simulink model "test_4"  (R2017b)
settings: Solver=VariableStepAuto  StartTime=0.0  StopTime=3  RelTol=1e-3
values from neighbouring files (symbols this model uses):
  Cwy1 = 0.0074    [Parameters (2).m]    (also in Parameters.m)
  Cwy2 = 0.0527    [Parameters (2).m]    (also in Parameters.m)
  Jyy = 0.78    [Parameters (2).m]    (also in Parameters.m)
  k1_k = 0.3    [Parameters (2).m]    (also in Parameters.m)
  k2_k = 0.16732    [Parameters (2).m]    (also in Parameters.m)
  K_thruster = 2.89    [Parameters (2).m]    (also in Parameters.m)
  kc = 57.2958    [Parameters (2).m]    (also in Parameters.m)
  lambda55 = 0.9    [Parameters (2).m]    (also in Parameters.m)
  T_thruster = 0.1    [Parameters (2).m]    (also in Parameters.m)
settings Model: Creator=Eugene  LastModifiedBy=Eugene

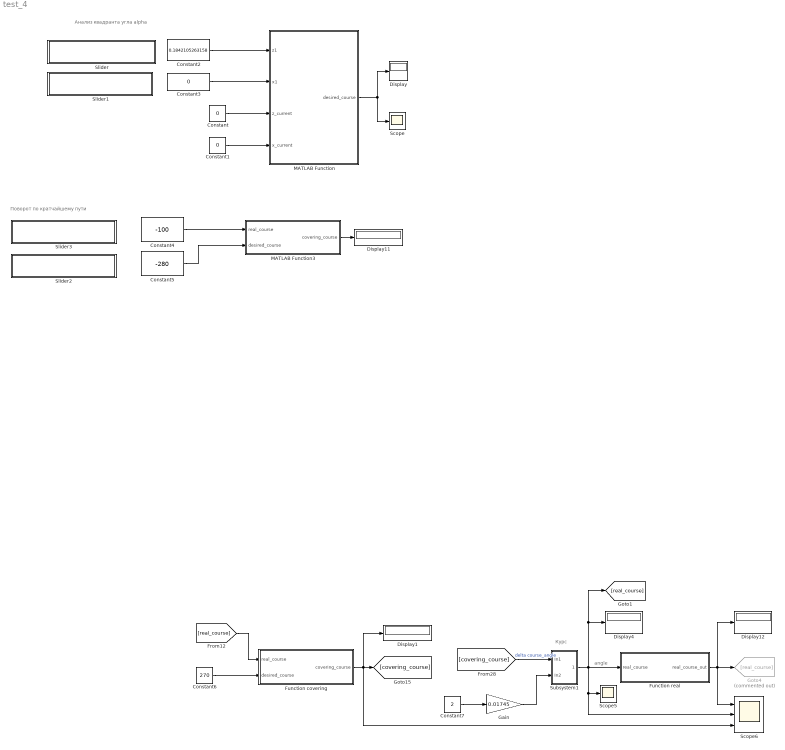
== system test_4 ==
  note: Поворот по кратчайшему пути
  note: Анализ квадранта угла alpha
  note: Курс
  note: angle
  Constant : Constant  Value=0
  Constant1 : Constant  Value=0
  Constant2 : Constant  Value=0.1842105263158
  Constant3 : Constant  Value=0
  Constant4 : Constant  Value=-100
  Constant5 : Constant  Value=-280
  Constant6 : Constant  Value=270
  Constant7 : Constant  Value=2
  Display{,1,4,11..12} (5 alike) : Display
  Function covering : MATLAB Function  TreatAsAtomicUnit=on
  Function real : MATLAB Function  TreatAsAtomicUnit=on
  Gain : Gain  Gain=0.01745
  Goto4 : Goto  Commented=on  GotoTag=real_course
  MATLAB Function : MATLAB Function  TreatAsAtomicUnit=on
  MATLAB Function3 : MATLAB Function  TreatAsAtomicUnit=on
  Scope : Scope
  Scope5 : Scope
  Scope6 : Scope  NumInputPorts=3
  Slider : Subsystem  DialogController=hmiCreateDDGDialog  IsWebBlock=on  mask(MWDashboardBlock){webBlockId=2d4f2b3b-9694-4286-a5f2-3185fd8971f2, webBlockType=slider, ShowInLibBrowser=on, ShowInitialText=on, HMISrcModelName=test_4}
      mask prompts: webBlockId "WebBlock Id"; webBlockType "WebBlock Type"; HMISrcModelName "Source Model"
      mask help: SimulinkHMI:dialogs:SliderDialogDesc
      mask Help: helpview([docroot '/mapfiles/simulink.map'], 'hmi_slider')
      mask Display:
      | if strcmp(get_param(bdroot(gcb),'BlockDiagramType'), 'library')
      |     image([(matlabroot) '/toolbox/simulink/hmi/icons/Slider.png']);
      | end
  Slider1 : Subsystem  DialogController=hmiCreateDDGDialog  IsWebBlock=on  mask(MWDashboardBlock){webBlockId=10c0b1f4-f331-46f9-accf-0d1c75457103, webBlockType=slider, ShowInLibBrowser=on, ShowInitialText=on, HMISrcModelName=test_4}
      mask prompts: webBlockId "WebBlock Id"; webBlockType "WebBlock Type"; HMISrcModelName "Source Model"
      mask help: SimulinkHMI:dialogs:SliderDialogDesc
      mask Help: helpview([docroot '/mapfiles/simulink.map'], 'hmi_slider')
      mask Display:
      | if strcmp(get_param(bdroot(gcb),'BlockDiagramType'), 'library')
      |     image([(matlabroot) '/toolbox/simulink/hmi/icons/Slider.png']);
      | end
  Slider2 : Subsystem  DialogController=hmiCreateDDGDialog  IsWebBlock=on  mask(MWDashboardBlock){webBlockId=beae14a9-6052-4aa7-916a-4f04d7c05d55, webBlockType=slider, ShowInLibBrowser=on, ShowInitialText=on, HMISrcModelName=test_4}
      mask prompts: webBlockId "WebBlock Id"; webBlockType "WebBlock Type"; HMISrcModelName "Source Model"
      mask help: SimulinkHMI:dialogs:SliderDialogDesc
      mask Help: helpview([docroot '/mapfiles/simulink.map'], 'hmi_slider')
      mask Display:
      | if strcmp(get_param(bdroot(gcb),'BlockDiagramType'), 'library')
      |     image([(matlabroot) '/toolbox/simulink/hmi/icons/Slider.png']);
      | end
  Slider3 : Subsystem  DialogController=hmiCreateDDGDialog  IsWebBlock=on  mask(MWDashboardBlock){webBlockId=003fc597-b61a-4663-9dbd-5e54f20fd45b, webBlockType=slider, ShowInLibBrowser=on, ShowInitialText=on, HMISrcModelName=test_4}
      mask prompts: webBlockId "WebBlock Id"; webBlockType "WebBlock Type"; HMISrcModelName "Source Model"
      mask help: SimulinkHMI:dialogs:SliderDialogDesc
      mask Help: helpview([docroot '/mapfiles/simulink.map'], 'hmi_slider')
      mask Display:
      | if strcmp(get_param(bdroot(gcb),'BlockDiagramType'), 'library')
      |     image([(matlabroot) '/toolbox/simulink/hmi/icons/Slider.png']);
      | end
  Subsystem1 : Subsystem
  wires:
  MATLAB Function/1(desired_course) -> Scope/1, Display/1
  Constant1/1 -> MATLAB Function/4(x_current)
  Constant/1 -> MATLAB Function/3(z_current)
  Constant2/1 -> MATLAB Function/1(z1)
  Constant3/1 -> MATLAB Function/2(x1)
  MATLAB Function3/1(covering_course) -> Display11/1
  Constant4/1 -> MATLAB Function3/1(real_course)
  Constant5/1 -> MATLAB Function3/2(desired_course)
  [real_course] -> Function covering/1(real_course)
  Function covering/1(covering_course) -> Scope6/3, Display1/1, [covering_course]
  Subsystem1/1(Out1) -> Scope6/2, Scope5/1, [real_course], Display4/1, Function real/1(real_course)
  [covering_course] -> Subsystem1/1(In1)  "delta course_angle"
  Function real/1(real_course_out) -> Scope6/1, Goto4/1, Display12/1
  Constant7/1 -> Gain/1
  Gain/1 -> Subsystem1/2(In2)
  Constant6/1 -> Function covering/2(desired_course)

== system test_4/Slider ==

== system test_4/Slider1 ==

== system test_4/Slider2 ==

== system test_4/Slider3 ==

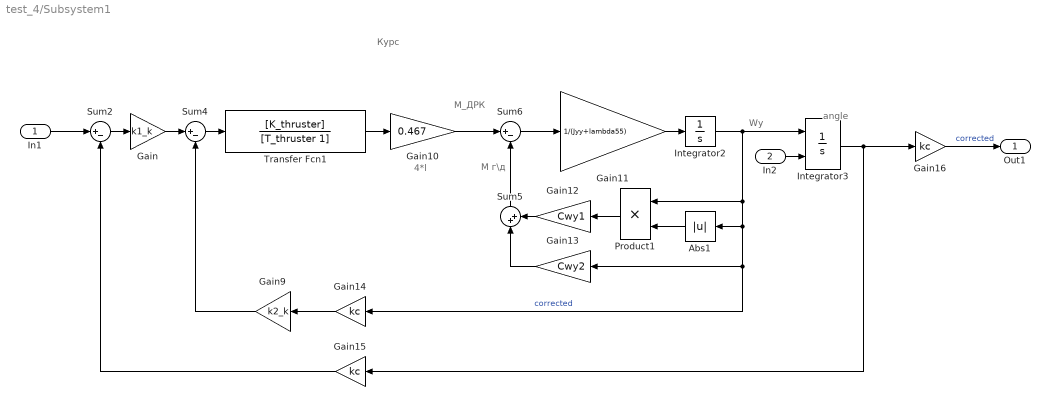
== system test_4/Subsystem1 ==
  note: Курс
  note: Wy
  note: M_ДРК
  note: 4*l
  note: angle
  note: M г\д
  In1 : Inport
  In2 : Inport  Port=2
  Abs1 : Abs
  Gain : Gain  Gain=k1_k
  Gain10 : Gain  Gain=0.467
  Gain11 : Gain  Gain=1/(Jyy+lambda55)
  Gain12 : Gain  Gain=Cwy1
  Gain13 : Gain  Gain=Cwy2
  Gain14 : Gain  Gain=kc
  Gain15 : Gain  Gain=kc
  Gain16 : Gain  Gain=kc
  Gain9 : Gain  Gain=k2_k
  Integrator2 : Integrator
  Integrator3 : Integrator  InitialConditionSource=external  InitialCondition=1.5708
  Product1 : Product
  Sum2 : Sum  Inputs=|+-
  Sum4 : Sum  Inputs=|+-
  Sum5 : Sum  Inputs=|++
  Sum6 : Sum  Inputs=|+-
  Transfer Fcn1 : TransferFcn  Numerator=[K_thruster]  Denominator=[T_thruster 1]
  Out1 : Outport
  wires:
  Gain12/1 -> Sum5/2
  Gain10/1 -> Sum6/1
  Product1/1 -> Gain12/1
  Gain11/1 -> Integrator2/1
  Gain9/1 -> Sum4/2
  Gain/1 -> Sum4/1
  Transfer Fcn1/1 -> Gain10/1
  Sum6/1 -> Gain11/1
  Gain14/1 -> Gain9/1
  Gain15/1 -> Sum2/2
  Gain13/1 -> Sum5/1
  Abs1/1 -> Product1/2
  Sum5/1 -> Sum6/2
  Integrator2/1 -> Gain14/1, Gain13/1, Abs1/1, Product1/1, Integrator3/1  "corrected"
  Sum2/1 -> Gain/1
  Integrator3/1 -> Gain16/1, Gain15/1
  Sum4/1 -> Transfer Fcn1/1
  In1/1 -> Sum2/1
  Gain16/1 -> Out1/1  "corrected"
  In2/1 -> Integrator3/2

== matlab function test_4/Function covering ==
  data: real_course input; desired_course input; covering_course output
function covering_course   = fcn(real_course, desired_course)

    % предстоит повернуться более чем на 180 градусов
    %if abs(desired_course - real_course) > 180
    %    covering_course = desired_course - 360 - real_course;
    %elseif desired_course < real_course
    %    covering_course = desired_course - real_course;
    %else    
    %    covering_course = desired_course;
    %end
    
    if abs(desired_course - real_course) > 180
        
        if desired_course > 180
            covering_course = desired_course - 360;
        elseif desired_course < -180
            covering_course = 360 + desired_course;
        else
            covering_course = desired_course;
        end
    else
        covering_course = desired_course;
    end
end

== matlab function test_4/MATLAB Function ==
  data: z1 input; x1 input; z_current input; desired_course output; x_current input
function desired_course = fcn(z1, x1, z_current, x_current)

delta_x = x1 - x_current;
delta_z = z1 - z_current;

if (delta_x >= 0) && (delta_z >= 0)
    desired_course = 57.2958*atan(delta_x / delta_z);
    
elseif (delta_x >= 0) && (delta_z < 0)
    desired_course = 180 - 57.2958*atan(delta_x / abs(delta_z));
    
elseif (delta_x < 0) && (delta_z <= 0)    
    desired_course = 180 + 57.2958*atan(abs(delta_x) / abs(delta_z));
    
elseif (delta_x < 0) && (delta_z > 0)    
    desired_course = 270 + 57.2958*atan(abs(delta_x) / delta_z);   
    
else 
    desired_course = -1;
   
end

== matlab function test_4/MATLAB Function3 ==
  data: real_course input; desired_course input; covering_course output
function covering_course   = fcn(real_course, desired_course)

    % Поворот по кратчайшему пути
    if abs(desired_course - real_course) > 180
        covering_course = desired_course - 360 - real_course;
    else
        covering_course = desired_course;
    end

end

== matlab function test_4/Function real ==
  data: real_course input; real_course_out output
function real_course_out   = fcn(real_course)

    % Приводим к стандарту
    if real_course < 0
        real_course_out = 360 - abs(real_course);
    elseif real_course >= 360
        real_course_out = real_course - 360;
    else    
        real_course_out = real_course;
    end

end
